simulink model "Arrays3_0"  (Simulink 8.7)
settings: Solver=FixedStepDiscrete  StartTime=0.0  StopTime=10000.0  RelTol=1e-3
settings Model: Creator=scaife  LastModifiedBy=hamza  ExtModeAutoUpdateStatusClock=off
settings DataIOCC: SignalLoggingSaveFormat=ModelDataLogs  SignalLoggingName=sigsOut
settings DebuggingCC: SaveWithParameterizedLinksMsg=none  SignalResolutionControl=TryResolveAllWithWarning  MultiTaskDSMMsg=warning  MultiTaskCondExecSysMsg=none
settings HardwareCC: TargetUnknown=on
settings SFSimCC: SimParseCustomCode=off
settings GRTTargetCC: GeneratePreprocessorConditionals=Use local settings  CombineOutputUpdateFcns=off  GRTInterface=on

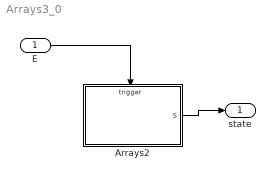
== system Arrays3_0 ==
  E : Inport
  Arrays2 : Stateflow chart  TreatAsAtomicUnit=on
  state : Outport
  wires:
  E/1 -> Arrays2/Trigger
  Arrays2/1(s) -> state/1

== stateflow chart Arrays2 ==
  state A/
    en:x[1][1][1]++
    x[1][1][1]+=2
    x[1][1][1]+=3
    x[1][1][1]=x[1][1][1]+1
    s = 1
  state B/
    en:x[1][1][1]++
    x[1][1][1]+=2
    x[1][1][1]+=3
    x[1][1][1]=x[1][1][1]+1
    s = 2
  state C/
    en:x[2][1][1]++
    x[2][1][1]+=2
    x[2][1][1]+=3
    x[2][1][1]=x[2][1][1]+1
    s = 3
  (default) -> A
  C -> A : E
  A -> B : E
  B -> C : E
  data: x local int32 size=3 2 2 [0..100] =1; s output int32
  events: E input RISING_EDGE_EVENT
